simulink model "data_collection_chemical_reactor"  (R2023b)
settings: Solver=VariableStepAuto  StartTime=0.0  StopTime=Tsim  RelTol=1e-3
values from neighbouring files (symbols this model uses):
  mag = 0.1    [chemical_reactor.m]
  Ts = 0.1    [chemical_reactor.m]
  x0 = (2*mx0).*rand(n+m,1)-mx0    [chemical_reactor.m]
settings Model: Creator=pietrotesi  LastModifiedBy=zjhu_
settings SolverCC: AlgebraicLoopSolver=TrustRegion
settings DataIOCC: ReturnWorkspaceOutputs=off
settings DebuggingCC: UnconnectedInputMsg=warning  UnconnectedOutputMsg=warning  UnconnectedLineMsg=warning
settings ModelReferenceCC: EnableRefExpFcnMdlSchedulingChecks=on
settings RTWCC: DLArmComputeVersion=19.05

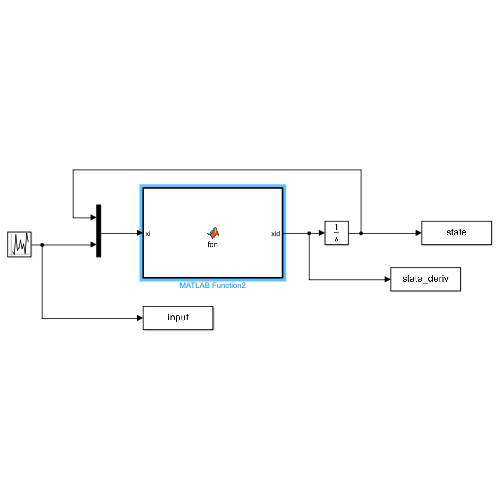
[thumbnail: Simulink's stored preview of the top-level diagram]
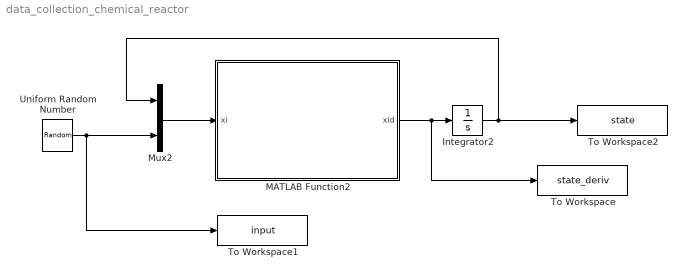
== system data_collection_chemical_reactor ==
  Integrator2 : Integrator  InitialCondition=x0
  MATLAB Function2 : MATLAB Function  TreatAsAtomicUnit=on
  Mux2 : Mux  Inputs=2
  To Workspace : ToWorkspace  VariableName=state_deriv  SaveFormat=Structure With Time  SampleTime=Ts
  To Workspace1 : ToWorkspace  VariableName=input  SaveFormat=Structure With Time  SampleTime=Ts
  To Workspace2 : ToWorkspace  VariableName=state  SaveFormat=Structure With Time  SampleTime=Ts
  Uniform Random Number : UniformRandomNumber  Minimum=-mag  Maximum=mag  SampleTime=Ts
  wires:
  Mux2/1 -> MATLAB Function2/1(xi)
  MATLAB Function2/1(xid) -> To Workspace/1, Integrator2/1
  Uniform Random Number/1 -> To Workspace1/1, Mux2/2
  Integrator2/1 -> To Workspace2/1, Mux2/1

== matlab function data_collection_chemical_reactor/MATLAB Function2 ==
  data: xi input; xid output
function xid = fcn(xi)
  
x1 = xi(1);
x2 = xi(2);
u = xi(3);
v  = xi(4);

xid = [4.25*x1 + x2 - 0.25*u - x1*u; -6.25*x1 - 2*x2; v];
